simulink model "Task_No3"  (R2023b)
settings: Solver=ode5  StartTime=0.0  StopTime=60*60*24  FixedStep=0.1  RelTol=1e-3
InitFcn:
  | PARAMETERS;
StartFcn:
  | PARAMETERS;
values from neighbouring files (symbols this model uses):
  Conv_C_to_K = 273.15    [PARAMETERS.m]
  P_CP_AIR = 1012    [PARAMETERS.m]
  P_HEATER_AIR_FLOW = 1    [PARAMETERS.m]
  T_HEATER = 50    [PARAMETERS.m]
  T_INIT_BDR = 20    [PARAMETERS.m]
  T_INIT_OUT = 2.9    [PARAMETERS.m]
libraries: fl_lib x9, nesl_utility x4
settings Model: Creator=Selim  LastModifiedBy=Selim

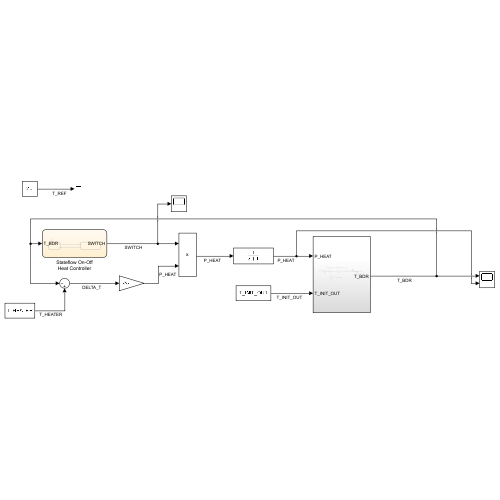
[thumbnail: Simulink's stored preview of the top-level diagram]
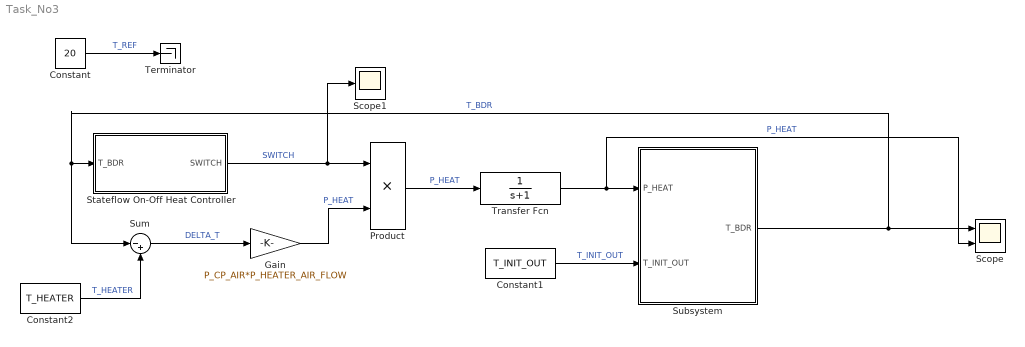
== system Task_No3 ==
  Constant : Constant  Value=20
  Constant1 : Constant  Value=T_INIT_OUT
  Constant2 : Constant  Value=T_HEATER
  Gain : Gain  Gain=P_CP_AIR*P_HEATER_AIR_FLOW
  Product : Product
  Scope : Scope  NumInputPorts=2
  Scope1 : Scope
  Stateflow On-Off Heat Controller : Stateflow chart  TreatAsAtomicUnit=on
  Subsystem : Subsystem
  Sum : Sum  Inputs=|-+
  Terminator : Terminator
  Transfer Fcn : TransferFcn  Denominator=[1 1]
  wires:
  Transfer Fcn/1 -> Scope/2, Subsystem/1(P_HEAT)  "P_HEAT"
  Constant1/1 -> Subsystem/2(T_INIT_OUT)  "T_INIT_OUT"
  Subsystem/1(T_BDR) -> Sum/1, Stateflow On-Off Heat Controller/1(T_BDR), Scope/1  "T_BDR"
  Constant/1 -> Terminator/1  "T_REF"
  Stateflow On-Off Heat Controller/1(SWITCH) -> Scope1/1, Product/1  "SWITCH"
  Product/1 -> Transfer Fcn/1  "P_HEAT"
  Sum/1 -> Gain/1  "DELTA_T"
  Constant2/1 -> Sum/2  "T_HEATER"
  Gain/1 -> Product/2  "P_HEAT"

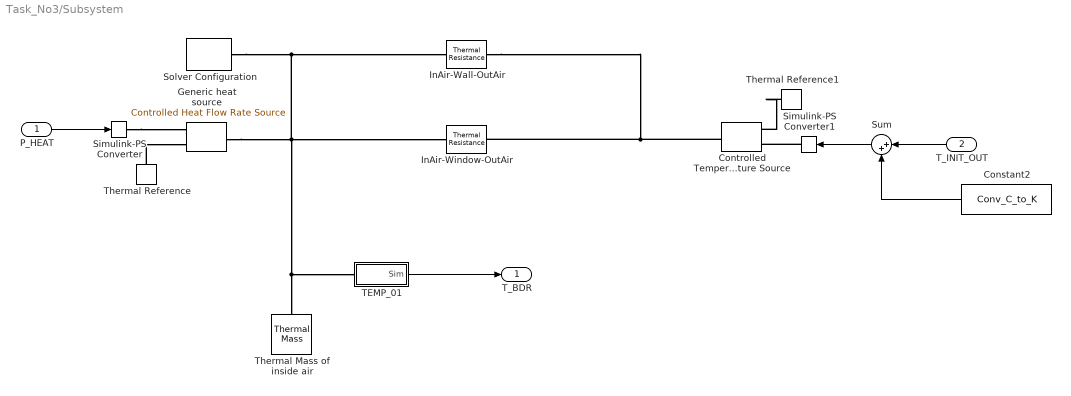
== system Task_No3/Subsystem ==
  P_HEAT : Inport
  T_INIT_OUT : Inport  Port=2
  Constant2 : Constant  Value=Conv_C_to_K
  Controlled Temperature Source : fl_lib/Thermal/Thermal Sources/Controlled Temperature Source
  Generic heat source : fl_lib/Thermal/Thermal Sources/Controlled Heat Flow Rate Source
  InAir-Wall-OutAir : fl_lib/Thermal/Thermal Elements/Thermal Resistance  resistance=R_WALL K/W  T_specify=off  T_priority=None  T=0 K  T_nominal_specify=off  T_nominal_unit=K  T_nominal_value=1  Q_specify=off  Q_priority=None  Q=0 W  Q_nominal_specify=off  Q_nominal_unit=W  Q_nominal_value=1
  InAir-Window-OutAir : fl_lib/Thermal/Thermal Elements/Thermal Resistance  resistance=R_WINDOW K/W  T_specify=off  T_priority=None  T=0 K  T_nominal_specify=off  T_nominal_unit=K  T_nominal_value=1  Q_specify=off  Q_priority=None  Q=0 W  Q_nominal_specify=off  Q_nominal_unit=W  Q_nominal_value=1
  Simulink-PS Converter : nesl_utility/Simulink-PS Converter  PhysicalDomain=network_engine_domain  SubClassName=ps_input  LeftPortType=input  RightPortType=output  PseudoPeriodic=off  Frequencies=[]  NoiseDistribution=none  NoiseParameters=[]  Unit=1  AffineConversion=off  FilteringAndDerivatives=provide  SimscapeFilterOrder=1  InputFilterTimeConstant=0.001  UdotUserProvided=0
  Simulink-PS Converter1 : nesl_utility/Simulink-PS Converter  PhysicalDomain=network_engine_domain  SubClassName=ps_input  LeftPortType=input  RightPortType=output  PseudoPeriodic=off  Frequencies=[]  NoiseDistribution=none  NoiseParameters=[]  Unit=1  AffineConversion=off  FilteringAndDerivatives=provide  SimscapeFilterOrder=1  InputFilterTimeConstant=0.001  UdotUserProvided=0
  Solver Configuration : nesl_utility/Solver Configuration  PhysicalDomain=network_engine_domain  SubClassName=solver  LeftPortType=input  RightPortType=generic  Tones=[]  Harmonics=[]  SimulateNoise=off  Profile=off  UseLocalSampling=off  EnableSwitchedLinearOptims=on  FrequencyDomain=off  UseCCode=off  RelTol=0.001  AbsTol=0.001  MinStep=1e-09  ToWorkspace=off  RevertToSquareIcSolve=off  NumHomotopyIterations=100  PhasorMode=off  PhasorModeNumHarmonics=1  ConsistencySolver=NEWTON_XTOL_AFTER_FTOL  IndexReductionMethod=DerivativeReplacement  DoDC=off  ResidualTolerance=1e-09  ConsistencyTolSource=GLOBAL  ConsistencyAbsTol=0.001  ConsistencyRelTol=0.001  ConsistencyTolFactor=0.001  UseLocalSolver=off  LocalSolverChoice=NE_BACKWARD_EULER_ADVANCER  ResolveIndetEquations=on  FunctionEvalNumThread=1  LocalSolverSampleTime=0.001  DoFixedCost=off  MaxNonlinIter=3  MaxModeIter=2  ComputeImpulses=off  ImpulseIterations=2  LinearAlgebra=auto  LinearAlgebraNumThread=0  EquationFormulation=NE_TIME_EF  DelaysMemoryBudget=1024  AutomaticFiltering=on  FilteringTimeConstant=0.001  PartitionStorageMethod=AS_NEEDED  PartitionMemoryBudget=1024  PartitionMethod=ROBUST  MultibodyUseLocalSolver=off  MultibodyLocalSolverChoice=ODE1  MultibodyLocalSolverSampleTime=0.001
  Sum : Sum  Inputs=|++
  TEMP_01 : Subsystem
  Thermal Mass of inside air : fl_lib/Thermal/Thermal Elements/Thermal Mass  mass_type=foundation.enum.constant_variable.constant  mass=P_M_AIR kg  sp_heat=P_CP_AIR J/(K*kg)  mass_min=1e-6 kg  num_ports=foundation.enum.numPorts2.one  m_specify=off  m_priority=High  m=1 kg  m_nominal_specify=off  m_nominal_unit=kg  m_nominal_value=1  T_specify=on  T_priority=High  T=T_INIT_BDR degC  T_nominal_specify=off  T_nominal_unit=K  T_nominal_value=1  Q_specify=off  Q_priority=None  Q=0 W  Q_nominal_specify=off  Q_nominal_unit=W  Q_nominal_value=1
  Thermal Reference : fl_lib/Thermal/Thermal Elements/Thermal Reference
  Thermal Reference1 : fl_lib/Thermal/Thermal Elements/Thermal Reference
  T_BDR : Outport
  wires:
  Constant2/1 -> Sum/2
  Sum/1 -> Simulink-PS Converter1/1
  TEMP_01/1(Sim) -> T_BDR/1
  P_HEAT/1 -> Simulink-PS Converter/1
  T_INIT_OUT/1 -> Sum/1
  connections:
  Thermal Reference/LConn1 -- Generic heat source/RConn2
  Controlled Temperature Source/LConn1 -- InAir-Wall-OutAir/RConn1 -- InAir-Window-OutAir/RConn1
  Generic heat source/LConn1 -- Solver Configuration/RConn1 -- InAir-Wall-OutAir/LConn1 -- InAir-Window-OutAir/LConn1 -- Thermal Mass of inside air/LConn1 -- TEMP_01/LConn1
  Thermal Reference1/LConn1 -- Controlled Temperature Source/RConn2
  Simulink-PS Converter/RConn1 -- Generic heat source/RConn1
  Simulink-PS Converter1/RConn1 -- Controlled Temperature Source/RConn1

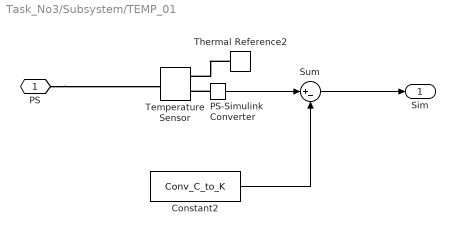
== system Task_No3/Subsystem/TEMP_01 ==
  Constant2 : Constant  Value=Conv_C_to_K
  PS-Simulink Converter : nesl_utility/PS-Simulink Converter  PhysicalDomain=network_engine_domain  SubClassName=ps_output  LeftPortType=input  RightPortType=output  PseudoPeriodic=off  Frequencies=[]  VectorFormat=inherit  Unit=inherit  AffineConversion=off
  Sum : Sum  Inputs=|+-
  Temperature Sensor : fl_lib/Thermal/Thermal Sensors/Temperature Sensor  temperature_measure=foundation.enum.MeasurementReference.difference
  Thermal Reference2 : fl_lib/Thermal/Thermal Elements/Thermal Reference
  PS : PMIOPort  Side=Left
  Sim : Outport
  wires:
  Sum/1 -> Sim/1
  PS-Simulink Converter/1 -> Sum/1
  Constant2/1 -> Sum/2
  connections:
  Thermal Reference2/LConn1 -- Temperature Sensor/RConn1
  PS-Simulink Converter/LConn1 -- Temperature Sensor/RConn2
  PS/RConn1 -- Temperature Sensor/LConn1

== stateflow chart Task_No3/Stateflow On-Off Heat Controller ==
  state Off
    entry:
    SWITCH = 0;
  state On
    entry:
    SWITCH = 1
  (default) -> Off
  Off -> On : [T_BDR<18]
  On -> Off : [T_BDR>22]
  data: T_BDR input; SWITCH output
